simulink model "Tank_Modell_Student"  (R2020b)
settings: Solver=ode45  StartTime=0.0  StopTime=1200  RelTol=1e-3
undefined symbols (not defined in the file or in its folder): parSys
settings Model: Creator=Wolfgang Kemmetmüller  LastModifiedBy=Armin Wessel
settings DataIOCC: LimitDataPoints=on  SaveFormat=Array  ReturnWorkspaceOutputs=off
settings OptimizationCC: BlockReduction=off  BooleanDataType=off  LifeSpan=inf
settings DebuggingCC: SaveWithParameterizedLinksMsg=none  UnderspecifiedInitializationDetection=Classic  MergeDetectMultiDrivingBlocksExec=none  SignalResolutionControl=TryResolveAllWithWarning  SFUnexpectedBacktrackingDiag=warning  SFNoUnconditionalDefaultTransitionDiag=warning  SFExecutionAtInitializationDiag=none  ArithmeticOperatorsInVariantConditions=warning
settings HardwareCC: ProdBitPerPointer=32  ProdBitPerSizeT=32  ProdBitPerPtrDiffT=32  ProdLargestAtomicFloat=None  ProdIntDivRoundTo=Undefined  ProdEndianess=Unspecified  ProdWordSize=32  ProdHWDeviceType=32-bit Generic  TargetUnknown=on
settings ModelReferenceCC: PropagateSignalLabelsOutOfModel=off
settings SFSimCC: SimUseLocalCustomCode=off  CustomCodeUndefinedFunction=UseInterfaceOnly
settings RTWCC: RTWUseLocalCustomCode=off
settings CodeAppCC: StateflowObjectComments=on
settings GRTTargetCC: TargetLangStandard=C89/C90 (ANSI)
settings ConfigComp: CovMetricSettings=dw  CovSaveCumulativeToWorkspaceVar=on  CovSaveSingleToWorkspaceVar=on  CovExternalEMLEnable=off

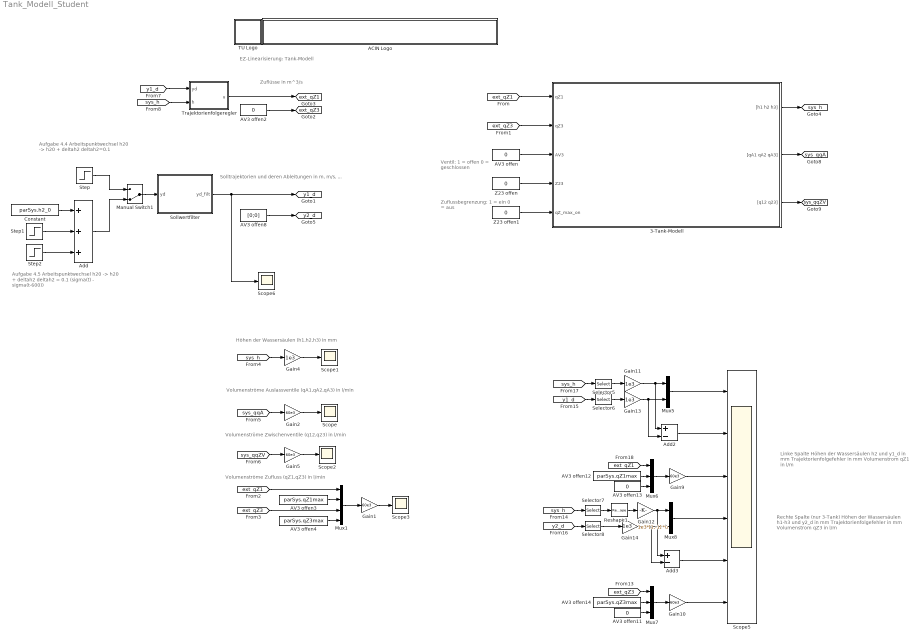
== system Tank_Modell_Student ==
  note: EZ-Linearisierung: Tank-Modell
  note: Höhen der Wassersäulen (h1,h2,h3) in mm
  note: Volumenströme Auslassventile (qA1,qA2,qA3) in l/min
  note: Volumenströme Zwischenventile (q12,q23) in l/min
  note: Ventil:
      | 1 = offen
      | 0 = geschlossen
  note: Volumenströme Zufluss (qZ1,qZ3) in l/min
  note: Linke Spalte
      | Höhen der Wassersäulen h2 und y1_d in mm
      | Trajektorienfolgefehler in mm
      | Volumenstrom qZ1 in l/m
  note: Zuflussbegrenzung:
      | 1 = ein
      | 0 = aus
  note: Rechte Spalte (nur 3-Tank)
      | Höhen der Wassersäulen h1-h3 und y2_d in mm
      | Trajektorienfolgefehler in mm
      | Volumenstrom qZ3 in l/m
  note: Zuflüsse in m^3/s
  note: Solltrajektorien und deren Ableitungen in m, m/s, ...
  note: Aufgabe 4.4 Arbeitspunktwechsel
      | h20 -> h20 + deltah2
      | deltah2=0.1
  note: Aufgabe 4.5 Arbeitspunktwechsel
      | h20 -> h20 + deltah2
      | deltah2 = 0.1 (sigma(t) - sigma(t-600))
  3-Tank-Modell : Subsystem
      mask init:
      | S = get_param(gcb,'UserData');
      mask Display:
      | image(S.pic);
      | port_label('input', 1, 'qZ1');
      | port_label('input', 2, 'qZ3');
      | port_label('input', 3, 'AV3');
      | port_label('input', 4, 'Z23');
      | port_label('input', 5, 'q_max_on');
      | port_label('output', 1, '[h1 h2 h3]');
      | port_label('output', 2, '[qA1 qA2 qA3]');
      | port_label('output', 3, '[q12 q23]');
  ACIN Logo : Subsystem
      mask init:
      | s = get_param(gcb,'UserData');
      mask Display:
      | image(s.logo,[0 0 439 45]);
      | %axis image
  AV3 offen{,2,11,13} (4 alike) : Constant  Value=0
  AV3 offen12 : Constant  Value=parSys.qZ1max  SampleTime=parSys.Ta
  AV3 offen14 : Constant  Value=parSys.qZ3max  SampleTime=parSys.Ta
  AV3 offen3 : Constant  Value=parSys.qZ1max  SampleTime=parSys.Ta
  AV3 offen4 : Constant  Value=parSys.qZ3max  SampleTime=parSys.Ta
  AV3 offen8 : Constant  Value=[0;0]
  Add : Sum  Inputs=+++
  Add2 : Sum  Inputs=+-
  Add3 : Sum  Inputs=+-
  Constant : Constant  Value=parSys.h2_0
  Gain{1..2,5,9..10} (5 alike) : Gain  Gain=60e3
  Gain{4,11,13..14} (4 alike) : Gain  Gain=1e3
  Gain12 : Gain  Gain=1e3*[1,-1]  Multiplication=Matrix(K*u)
  Manual Switch1 : ManualSwitch  CurrentSetting=0
  Mux1 : Mux
  Mux5 : Mux  Inputs=2
  Mux6 : Mux  Inputs=3
  Mux7 : Mux  Inputs=3
  Mux8 : Mux  Inputs=2
  Reshape1 : Reshape  OutputDimensionality=Column vector (2-D)
  Scope{,1..3,6} (5 alike) : Scope
  Scope5 : Scope  NumInputPorts=6
  Selector5 : Selector  InputPortWidth=3  IndexOptions=Index vector (dialog)  Indices=[2]  OutputSizes=1
  Selector6 : Selector  InputPortWidth=3  IndexOptions=Index vector (dialog)  Indices=[1]  OutputSizes=1
  Selector7 : Selector  InputPortWidth=3  IndexOptions=Index vector (dialog)  Indices=[1 3]  OutputSizes=1
  Selector8 : Selector  InputPortWidth=2  IndexOptions=Index vector (dialog)  Indices=[1]  OutputSizes=1
  Sollwertfilter : MATLAB Function  TreatAsAtomicUnit=on
  Step : Step  Before=parSys.h2_0  After=parSys.h2_0+parSys.deltah2  SampleTime=0
  Step1 : Step  Time=0  After=0.1  SampleTime=0
  Step2 : Step  Time=600  After=-0.1  SampleTime=0
  TU Logo : Subsystem
      mask init:
      | s = get_param(gcb,'UserData');
      mask Display: image(s.logo,[0 0 45 45]);
  Trajektorienfolgeregler : MATLAB Function  TreatAsAtomicUnit=on
  Z23 offen : Constant  Value=0
  Z23 offen1 : Constant  Value=0
  tag scope: ext_qZ1=global, ext_qZ3=global, sys_h=global, sys_qqA=global, sys_qqZV=global, y1_d=global, y2_d=global
  wires:
  [sys_qqA] -> Gain2/1
  [sys_qqZV] -> Gain5/1
  [sys_h] -> Gain4/1
  3-Tank-Modell/3("[q12 q23]") -> [sys_qqZV]
  3-Tank-Modell/2("[qA1 qA2 qA3]") -> [sys_qqA]
  AV3 offen/1 -> 3-Tank-Modell/3(AV3)
  Z23 offen/1 -> 3-Tank-Modell/4(Z23)
  [ext_qZ1] -> 3-Tank-Modell/1(qZ1)
  [ext_qZ3] -> 3-Tank-Modell/2(qZ3)
  AV3 offen2/1 -> [ext_qZ3]
  [ext_qZ1] -> Mux1/1
  [ext_qZ3] -> Mux1/3
  AV3 offen3/1 -> Mux1/2
  AV3 offen4/1 -> Mux1/4
  Gain5/1 -> Scope2/1
  Gain2/1 -> Scope/1
  Gain4/1 -> Scope1/1
  Mux1/1 -> Gain1/1
  Gain1/1 -> Scope3/1
  Sollwertfilter/1(yd_filt) -> Scope6/1, [y1_d]
  Z23 offen1/1 -> 3-Tank-Modell/5(qZ_max_on)
  AV3 offen8/1 -> [y2_d]
  [ext_qZ3] -> Mux7/1
  Selector6/1 -> Gain13/1
  Mux7/1 -> Gain10/1
  AV3 offen11/1 -> Mux7/3
  [sys_h] -> Selector7/1
  AV3 offen14/1 -> Mux7/2
  [ext_qZ1] -> Mux6/1
  Selector7/1 -> Reshape1/1
  Reshape1/1 -> Gain12/1
  [y2_d] -> Selector8/1
  Gain14/1 -> Mux8/2, Add3/2
  [sys_h] -> Selector5/1
  [y1_d] -> Selector6/1
  AV3 offen12/1 -> Mux6/2
  AV3 offen13/1 -> Mux6/3
  Selector8/1 -> Gain14/1
  Gain11/1 -> Add2/1, Mux5/1
  Add3/1 -> Scope5/5
  Mux6/1 -> Gain9/1
  Gain9/1 -> Scope5/3
  Selector5/1 -> Gain11/1
  Mux5/1 -> Scope5/1
  Add2/1 -> Scope5/2
  Gain13/1 -> Add2/2, Mux5/2
  Gain12/1 -> Mux8/1, Add3/1
  Mux8/1 -> Scope5/4
  Gain10/1 -> Scope5/6
  [sys_h] -> Trajektorienfolgeregler/2(h)
  [y1_d] -> Trajektorienfolgeregler/1(yd)
  Trajektorienfolgeregler/1(u) -> [ext_qZ1]
  Manual Switch1/1 -> Sollwertfilter/1(yd)
  Step/1 -> Manual Switch1/1
  Add/1 -> Manual Switch1/2
  Constant/1 -> Add/1
  Step1/1 -> Add/2
  Step2/1 -> Add/3
  3-Tank-Modell/1("[h1 h2 h3]") -> [sys_h]

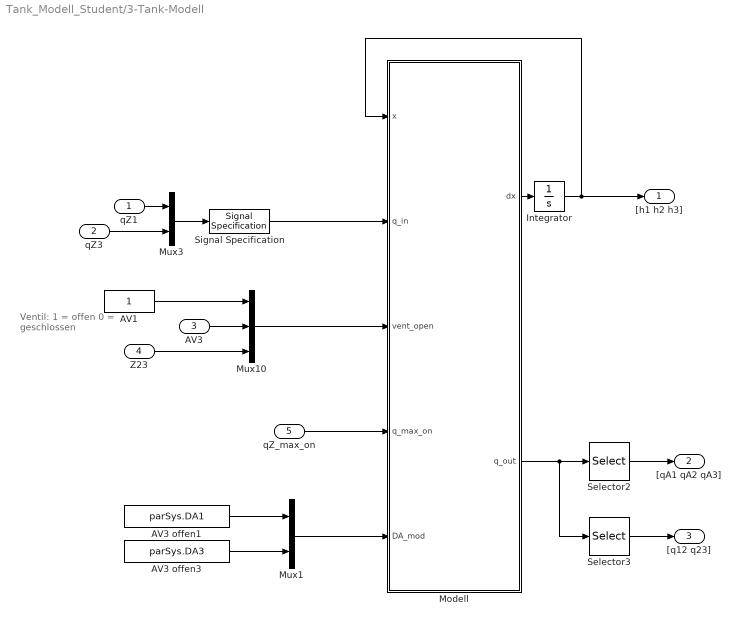
== system Tank_Modell_Student/3-Tank-Modell ==
  note: Ventil:
      | 1 = offen
      | 0 = geschlossen
  qZ1 : Inport
  qZ3 : Inport  Port=2
  AV3 : Inport  Port=3
  Z23 : Inport  Port=4
  qZ_max_on : Inport  Port=5
  AV1 : Constant
  AV3 offen1 : Constant  Value=parSys.DA1
  AV3 offen3 : Constant  Value=parSys.DA3
  Integrator : Integrator  InitialCondition=[parSys.h1_0;parSys.h2_0;parSys.h3_0]
  Modell : MATLAB Function  TreatAsAtomicUnit=on
  Mux1 : Mux  Inputs=2
  Mux10 : Mux  Inputs=3
  Mux3 : Mux  Inputs=2
  Selector2 : Selector  InputPortWidth=5  IndexOptions=Index vector (dialog)  Indices=[1 2 3]  OutputSizes=1
  Selector3 : Selector  InputPortWidth=5  IndexOptions=Index vector (dialog)  Indices=[4 5]  OutputSizes=1
  Signal Specification : SignalSpecification  Dimensions=2
  "[h1 h2 h3]" : Outport  VectorParamsAs1DForOutWhenUnconnected=off
  "[qA1 qA2 qA3]" : Outport  Port=2  VectorParamsAs1DForOutWhenUnconnected=off
  "[q12 q23]" : Outport  Port=3  VectorParamsAs1DForOutWhenUnconnected=off
  wires:
  AV1/1 -> Mux10/1
  qZ1/1 -> Mux3/1
  qZ3/1 -> Mux3/2
  Modell/2(q_out) -> Selector3/1, Selector2/1
  Selector2/1 -> "[qA1 qA2 qA3]"/1
  Selector3/1 -> "[q12 q23]"/1
  Z23/1 -> Mux10/3
  AV3/1 -> Mux10/2
  Mux10/1 -> Modell/3(vent_open)
  Mux3/1 -> Signal Specification/1
  Modell/1(dx) -> Integrator/1
  Integrator/1 -> Modell/1(x), "[h1 h2 h3]"/1
  Mux1/1 -> Modell/5(DA_mod)
  qZ_max_on/1 -> Modell/4(q_max_on)
  AV3 offen1/1 -> Mux1/1
  AV3 offen3/1 -> Mux1/2
  Signal Specification/1 -> Modell/2(q_in)

== system Tank_Modell_Student/ACIN Logo ==

== system Tank_Modell_Student/TU Logo ==

== matlab function Tank_Modell_Student/Trajektorienfolgeregler ==
  data: u output; yd input; h input; parSys parameter
function u = fcn(yd,h, parSys)

    %% Zustandszuweisung
    h1 = h(1);
    h2 = h(2);
    
    %% Parameterübergabe    
    Atank      = parSys.Atank;         % Grundfläche Tank
    rho         = parSys.rho;           % Dichte Wasser
    eta         = parSys.eta;           % Dynamische Viskosität Wasser
    g           = parSys.g;             % Gravitationskonstante
    alphaA1     = parSys.alphaA1;       % Kontraktionskoeffizient AV1
    DA1         = parSys.DA1;           % Durchmesser AV1
    alphaA2     = parSys.alphaA2;       % Kontraktionskoeffizient AV2
    AA2         = parSys.A2;            % Querschnittsflaeche AV2
    alphaA3     = parSys.alphaA3;       % Kontraktionskoeffizient AV3
    DA3         = parSys.DA3;           % Durchmesser AV3
    alpha120    = parSys.alpha12_0;     % Kontraktionskoeffizient ZV12
    A12         = parSys.A12;           % Querschnittsflaeche ZV12
    Dh12        = parSys.Dh12;          % hydraulischer Durchmesser
    lambdac12   = parSys.lambdac12;     % kritische Fliesszahl ZV12

    
    %% Reglerparameter
    a0 = parSys.a0;
    a1 = parSys.a1;
    deltah12 = parSys.deltah12
    
    %% Regler
    % qA1(h1,h2) und qA2(h1,h2)
    % aus Maple importiert
    qA1 = alphaA1 * DA1 ^ 2 * pi * sqrt(0.2e1) * sqrt(g) * sqrt(h1) / 0.4e1;
    qA2 = alphaA2 * AA2 * sqrt(0.2e1) * sqrt(g) * sqrt(h2);
    
    % Ableitungen von qA1(h1,h2) und qA2(h1,h2)
    % aus Maple importiert
    dqA1dh1 = alphaA1 * DA1 ^ 2 * pi * sqrt(0.2e1) * sqrt(g) * h1 ^ (-0.1e1 / 0.2e1) / 0.8e1;
    dqA1dh2 = 0;
    
    dqA2dh1 = 0;
    dqA2dh2 = alphaA2 * AA2 * sqrt(0.2e1) * sqrt(g) * h2 ^ (-0.1e1 / 0.2e1) / 0.2e1;
    
    % Fallunterscheidung
    if (h1 - h2) > deltah12
        q12 = alpha120 * tanh(0.2e1 * Dh12 * rho / eta * sqrt(0.2e1) * sqrt(g) * sqrt(h1 - h2) / lambdac12) * A12 * sqrt(0.2e1) * sqrt(g) * sqrt(h1 - h2);
        dq12dh1 = 0.2e1 * alpha120 * Dh12 * rho / eta * g / lambdac12 * (0.1e1 - tanh(0.2e1 * Dh12 * rho / eta * sqrt(0.2e1) * sqrt(g) * sqrt(h1 - h2) / lambdac12) ^ 2) * A12 + alpha120 * tanh(0.2e1 * Dh12 * rho / eta * sqrt(0.2e1) * sqrt(g) * sqrt(h1 - h2) / lambdac12) * A12 * sqrt(0.2e1) * sqrt(g) * (h1 - h2) ^ (-0.1e1 / 0.2e1) / 0.2e1;
        dq12dh2 = -0.2e1 * alpha120 * Dh12 * rho / eta * g / lambdac12 * (0.1e1 - tanh(0.2e1 * Dh12 * rho / eta * sqrt(0.2e1) * sqrt(g) * sqrt(h1 - h2) / lambdac12) ^ 2) * A12 - alpha120 * tanh(0.2e1 * Dh12 * rho / eta * sqrt(0.2e1) * sqrt(g) * sqrt(h1 - h2) / lambdac12) * A12 * sqrt(0.2e1) * sqrt(g) * (h1 - h2) ^ (-0.1e1 / 0.2e1) / 0.2e1;
    elseif (h1 - h2) < -deltah12
        q12 = -alpha120 * tanh(0.2e1 * Dh12 * rho / eta * sqrt(0.2e1) * sqrt(g) * sqrt(h2 - h1) / lambdac12) * A12 * sqrt(0.2e1) * sqrt(g) * sqrt(h2 - h1);
        dq12dh1 = 0.2e1 * alpha120 * Dh12 * rho / eta * g / lambdac12 * (0.1e1 - tanh(0.2e1 * Dh12 * rho / eta * sqrt(0.2e1) * sqrt(g) * sqrt(h2 - h1) / lambdac12) ^ 2) * A12 + alpha120 * tanh(0.2e1 * Dh12 * rho / eta * sqrt(0.2e1) * sqrt(g) * sqrt(h2 - h1) / lambdac12) * A12 * sqrt(0.2e1) * sqrt(g) * (h2 - h1) ^ (-0.1e1 / 0.2e1) / 0.2e1;
        dq12dh2 = -0.2e1 * alpha120 * Dh12 * rho / eta * g / lambdac12 * (0.1e1 - tanh(0.2e1 * Dh12 * rho / eta * sqrt(0.2e1) * sqrt(g) * sqrt(h2 - h1) / lambdac12) ^ 2) * A12 - alpha120 * tanh(0.2e1 * Dh12 * rho / eta * sqrt(0.2e1) * sqrt(g) * sqrt(h2 - h1) / lambdac12) * A12 * sqrt(0.2e1) * sqrt(g) * (h2 - h1) ^ (-0.1e1 / 0.2e1) / 0.2e1;
    else % approximierte Bereich -> Maple Herleitung
        dq120 = 4 * alpha120 * A12 * Dh12 * rho * g / eta / lambdac12;
        dq12_ddeltah12 = 0.2e1 * alpha120 * Dh12 * rho / eta * g / lambdac12 * (0.1e1 - tanh(0.2e1 * Dh12 * rho / eta * sqrt(0.2e1) * sqrt(g) * sqrt(deltah12) / lambdac12) ^ 2) * A12 + alpha120 * tanh(0.2e1 * Dh12 * rho / eta * sqrt(0.2e1) * sqrt(g) * sqrt(deltah12) / lambdac12) * A12 * sqrt(0.2e1) * sqrt(g) * deltah12 ^ (-0.1e1 / 0.2e1) / 0.2e1;
        % Steigung berechnen
        k = (dq12_ddeltah12 - dq120)/deltah12;
        dq12dh1 = k*abs(h1-h2)+dq120;
        dq12dh2 =-k*abs(h1-h2)-dq120;
        if h1 > h2
            q12 = alpha120 * tanh(0.2e1 * Dh12 * rho / eta * sqrt(0.2e1) * sqrt(g) * sqrt(h1 - h2) / lambdac12) * A12 * sqrt(0.2e1) * sqrt(g) * sqrt(h1 - h2);
        else
            q12 = -alpha120 * tanh(0.2e1 * Dh12 * rho / eta * sqrt(0.2e1) * sqrt(g) * sqrt(h2 - h1) / lambdac12) * A12 * sqrt(0.2e1) * sqrt(g) * sqrt(h2 - h1);
        end
    end
    
    Lfh = 0.1e1 / Atank * (q12 - qA2);
    Lf2h = -0.1e1 / Atank ^ 2 * (dq12dh1 - dqA2dh1) * (q12 + qA1) + 0.1e1 / Atank ^ 2 * (dq12dh2 - dqA2dh2) * (q12 - qA2);
    LgLfh = 0.1e1 / Atank ^ 2 * (dq12dh1 - dqA2dh1);
    
   u = 1/LgLfh *(yd(3) - Lf2h - a0*(h2-yd(1))- a1 * (Lfh-yd(2)));

end

== matlab function Tank_Modell_Student/Sollwertfilter ==
  data: yd_filt output; yd input; parSys parameter
function yd_filt = Filter(yd, parSys)
persistent x
if isempty(x) x=parSys.x0; end

yd_filt = parSys.C*x;
x  = parSys.A*x + parSys.b*yd;
end

== matlab function Tank_Modell_Student/3-Tank-Modell/Modell ==
  data: dx output; x input; q_in input; vent_open input; q_max_on input; DA_mod input; q_out output; parSys parameter
function [dx,q_out] = fcn(x,q_in,vent_open,q_max_on,DA_mod,parSys)
%#codegen

[dx,q_out] = Wassertank_mfun(x,q_in,vent_open,q_max_on,DA_mod,parSys);


% Function end
end
